simulink model "CG_5L_Inverter_simulinkblocks"  (R2024b)
settings: Solver=VariableStepAuto  StartTime=0.0  StopTime=0.6  RelTol=1e-3
libraries: spsIGBTDiodeLib x6, simulink x4, spsSeriesRLCBranchLib x4, spsDiodeLib x2, spsVoltageMeasurementLib x2, spsACVoltageSourceLib x1, spsDCVoltageSourceLib x1, spsCurrentMeasurementLib x1, spsRMSLib x1, sps_lib x1
settings Model: Creator=Kan  LastModifiedBy=DELL
settings SolverCC: AlgebraicLoopSolver=TrustRegion
settings DebuggingCC: ArithmeticOperatorsInVariantConditions=warning
settings SFSimCC: CustomCodeUndefinedFunction=UseInterfaceOnly
settings RTWCC: GPUComputeCapability=3.5

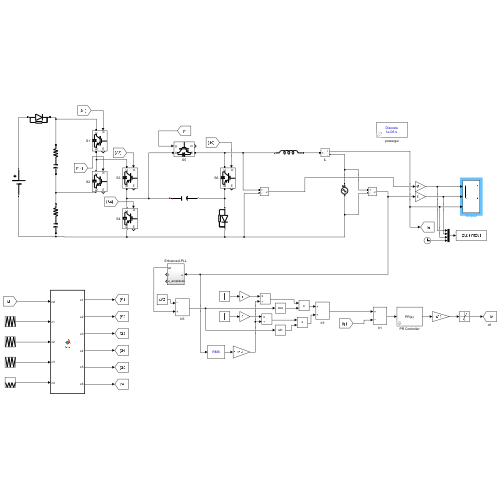
[thumbnail: Simulink's stored preview of the top-level diagram]
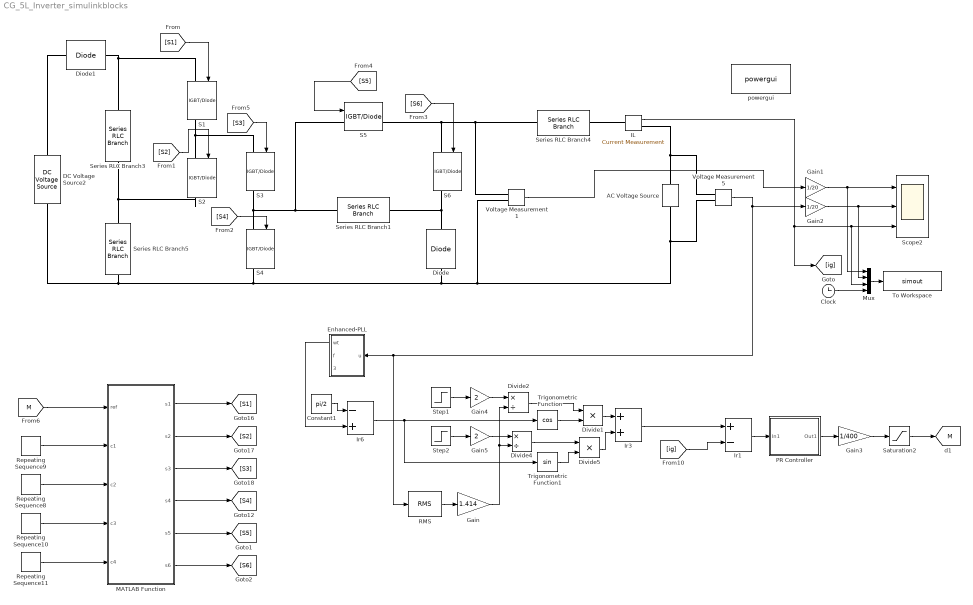
== system CG_5L_Inverter_simulinkblocks ==
  AC Voltage Source : spsACVoltageSourceLib/AC Voltage Source  Amplitude=325  Phase=0  Frequency=50  SampleTime=0  Measurements=None  BusType=swing  Pref=10e3  Qref=0  Qmin=-inf  Qmax=+inf
  Clock : Clock
  Constant1 : Constant  Value=pi/2
  DC Voltage Source2 : spsDCVoltageSourceLib/DC Voltage Source  Amplitude=400  Measurements=None
  Diode : spsDiodeLib/Diode  Ron=0.001  Lon=0  Vf=0.8  IC=0  UseSnubber=0  Rs=500000  Cs=250e-9  Measurements=off
  Diode1 : spsDiodeLib/Diode  Ron=0.001  Lon=0  Vf=0.8  IC=0  UseSnubber=0  Rs=500000  Cs=250e-9  Measurements=off
  Divide1 : Product  Inputs=**
  Divide2 : Product  Inputs=*/
  Divide4 : Product  Inputs=*/
  Divide5 : Product  Inputs=**
  Enhanced-PLL : Subsystem
  Gain : Gain  Gain=1.414
  Gain1 : Gain  Gain=1/20
  Gain2 : Gain  Gain=1/20
  Gain3 : Gain  Gain=1/400
  Gain4 : Gain  Gain=2
  Gain5 : Gain  Gain=2
  IL : spsCurrentMeasurementLib/Current Measurement  PhasorSimulation=off  OutputType=Complex  PSBequivalent=0
  Ir1 : Sum  Inputs=+-
  Ir3 : Sum
  Ir6 : Sum  Inputs=-+
  MATLAB Function : MATLAB Function  TreatAsAtomicUnit=on
  Mux : Mux
  PR Controller : Subsystem  mask(PR Controller){kp=5, kr=2000, f=50}
      mask prompts: kp "Proportional Gain (kp)"; kr "Resonant Gain (kr)"; f "Resonant Frequency (Hz)"
      mask help:
      | This block implements a Proportional Resonant Controller using transfer function kr*s / s^2+(2*pi*f)^2
      | It allows user to set the proportional gain (kp), resonant gain (kr) and resonant frequency in (Hz).
      |
      | Developed by Rodney Tan
      | Version 1.0 (Oct 2022)
      mask Display: disp('PR(s)');
  RMS : spsRMSLib/RMS  TrueRMS=on  Freq=50  RMSInit=120  Ts=0
  Repeating Sequence10 : simulink/Sources/Repeating Sequence  rep_seq_t=[0 1/20000 1/10000]  rep_seq_y=[0 -0.5 0]
  Repeating Sequence11 : simulink/Sources/Repeating Sequence  rep_seq_t=[0 1/20000 1/10000]  rep_seq_y=[-0.5 -1 -0.5]
  Repeating Sequence8 : simulink/Sources/Repeating Sequence  rep_seq_t=[0 1/20000 1/10000]  rep_seq_y=[0 0.5 0]
  Repeating Sequence9 : simulink/Sources/Repeating Sequence  rep_seq_t=[0 1/20000 1/10000]  rep_seq_y=[0.5 1 0.5]
  S{1..6} (6 alike) : spsIGBTDiodeLib/IGBT//Diode  Ron=1e-3  Rs=1e5  Cs=inf  Measurements=on
  Saturation2 : Saturate  UpperLimit=2  LowerLimit=-2  LinearizeAsGain=off
  Scope2 : Scope  NumInputPorts=3
  Series RLC Branch1 : spsSeriesRLCBranchLib/Series RLC Branch  LConnTagsString=__new0  RConnTagsString=__new0  BranchType=C  Resistance=1  Inductance=2e-3  SetiL0=off  InitialCurrent=0  Capacitance=4000e-6  Setx0=off  InitialVoltage=50  Measurements=None
  Series RLC Branch3 : spsSeriesRLCBranchLib/Series RLC Branch  LConnTagsString=__new0  RConnTagsString=__new0  BranchType=RC  Resistance=0.0002  Inductance=2e-3  SetiL0=off  InitialCurrent=0  Capacitance=2000e-6  Setx0=on  InitialVoltage=100  Measurements=None
  Series RLC Branch4 : spsSeriesRLCBranchLib/Series RLC Branch  LConnTagsString=__new0  RConnTagsString=__new0  BranchType=L  Resistance=0.0002  Inductance=6e-3  SetiL0=off  InitialCurrent=0  Capacitance=1e-6  Setx0=off  InitialVoltage=0  Measurements=None
  Series RLC Branch5 : spsSeriesRLCBranchLib/Series RLC Branch  LConnTagsString=__new0  RConnTagsString=__new0  BranchType=RC  Resistance=0.0002  Inductance=2e-3  SetiL0=off  InitialCurrent=0  Capacitance=2000e-6  Setx0=on  InitialVoltage=100  Measurements=None
  Step1 : Step  Time=0.3  Before=1000  After=0  SampleTime=0
  Step2 : Step  Time=0.3  After=1200  SampleTime=0
  To Workspace : ToWorkspace  VariableName=simout  SampleTime=-1
      settings: Save2DSignal=2-D array (concatenate along first dimension)
  Trigonometric Function : Trigonometry  Operator=cos
  Trigonometric Function1 : Trigonometry
  Voltage Measurement1 : spsVoltageMeasurementLib/Voltage Measurement  PhasorSimulation=off  OutputType=Complex  PSBequivalent=0
  Voltage Measurement5 : spsVoltageMeasurementLib/Voltage Measurement  PhasorSimulation=off  OutputType=Complex  PSBequivalent=0
  powergui : sps_lib/powergui  Priority=1  SimulationMode=Discrete  SampleTime=1e-6  frequency=60  Iterations=50  frequencyindice=0  Pbase=100e6  ErrMax=1e-4  UnitsV=kV  UnitsW=MW  buscounter=0  FunctionMessages=off  echomessages=off  EnableUseOfTLC=off  CurrentSourceSwitches=off  DisableSnubberDevices=off  DisableRonSwitches=off  DisableVfSwitches=off  DisplayEquations=off  AutomaticDiscreteSolvers=off  SolverType=Tustin/Backward Euler (TBE)  Interpol=off  ExternalGateDelay=off  methode=off  Ts=100  x0status=blocks  SPID=on  SwTol=0  HookPort=off  NonlinearTolerance=1e-4  nMaxIteration=100  ContinueOnMaxIteration=off  RestoreLinks=warning  ResistiveCurrentMeasurement=off  Frange=[0:2:500]  Ylog=off  Xlog=on  ShowGrid=off  save=off  variable=ZData  structure=0  ZoomFFT=off  StartTime=0.0  cycles=1  DisplayStyle=1  fundamental=60  FreqAxis=off  MaxFrequency=1000  frequencyindicesteady=1  RmsSteady=1  display=off
  tag scope: M=global
  wires:
  [S1] -> S1/1
  [S2] -> S2/1
  MATLAB Function/1(s1) -> [S1]
  MATLAB Function/4(s4) -> [S4]
  MATLAB Function/2(s2) -> [S2]
  [S3] -> S3/1
  [S4] -> S4/1
  [S5] -> S5/1
  [S6] -> S6/1
  MATLAB Function/5(s5) -> [S5]
  MATLAB Function/6(s6) -> [S6]
  Repeating Sequence11/1 -> MATLAB Function/5(c4)
  Repeating Sequence10/1 -> MATLAB Function/4(c3)
  Repeating Sequence8/1 -> MATLAB Function/3(c2)
  Repeating Sequence9/1 -> MATLAB Function/2(c1)
  Voltage Measurement1/1 -> Gain1/1
  Voltage Measurement5/1 -> RMS/1, Enhanced-PLL/1(u), Gain2/1
  Gain1/1 -> Mux/1, Scope2/1
  Gain2/1 -> Mux/2, Scope2/2
  Ir3/1 -> Ir1/1
  [ig] -> Ir1/2
  PR Controller/1(Out1) -> Gain3/1
  Saturation2/1 -> [M]
  Trigonometric Function1/1 -> Divide5/2
  Gain4/1 -> Divide2/1
  Divide5/1 -> Ir3/2
  Step2/1 -> Gain5/1
  Divide2/1 -> Divide1/1
  Constant1/1 -> Ir6/1
  Gain/1 -> Divide4/2, Divide2/2
  Gain5/1 -> Divide4/1
  Divide1/1 -> Ir3/1
  Step1/1 -> Gain4/1
  Trigonometric Function/1 -> Divide1/2
  RMS/1 -> Gain/1
  Ir6/1 -> Trigonometric Function1/1, Trigonometric Function/1
  Divide4/1 -> Divide5/1
  Enhanced-PLL/1(wt) -> Ir6/2
  Gain3/1 -> Saturation2/1
  Ir1/1 -> PR Controller/1(In1)
  IL/1 -> [ig], Mux/3, Scope2/3
  MATLAB Function/3(s3) -> [S3]
  [M] -> MATLAB Function/1(ref)
  Mux/1 -> To Workspace/1
  Clock/1 -> Mux/4
  connections:
  DC Voltage Source2/RConn1 -- Diode1/LConn1
  S5/RConn1 -- S6/LConn1 -- Series RLC Branch4/LConn1 -- Voltage Measurement1/LConn1
  S6/RConn1 -- Diode/LConn1 -- Series RLC Branch1/RConn1
  Voltage Measurement1/LConn2 -- DC Voltage Source2/LConn1 -- Series RLC Branch5/RConn1 -- S4/RConn1 -- Diode/RConn1 -- AC Voltage Source/LConn1 -- Voltage Measurement5/LConn2
  Series RLC Branch5/LConn1 -- S2/RConn1 -- Series RLC Branch3/RConn1
  S2/LConn1 -- S3/LConn1 -- S1/RConn1
  S4/LConn1 -- S5/LConn1 -- Series RLC Branch1/LConn1 -- S3/RConn1
  IL/LConn1 -- Series RLC Branch4/RConn1
  IL/RConn1 -- Voltage Measurement5/LConn1 -- AC Voltage Source/RConn1
  S1/LConn1 -- Diode1/RConn1 -- Series RLC Branch3/LConn1

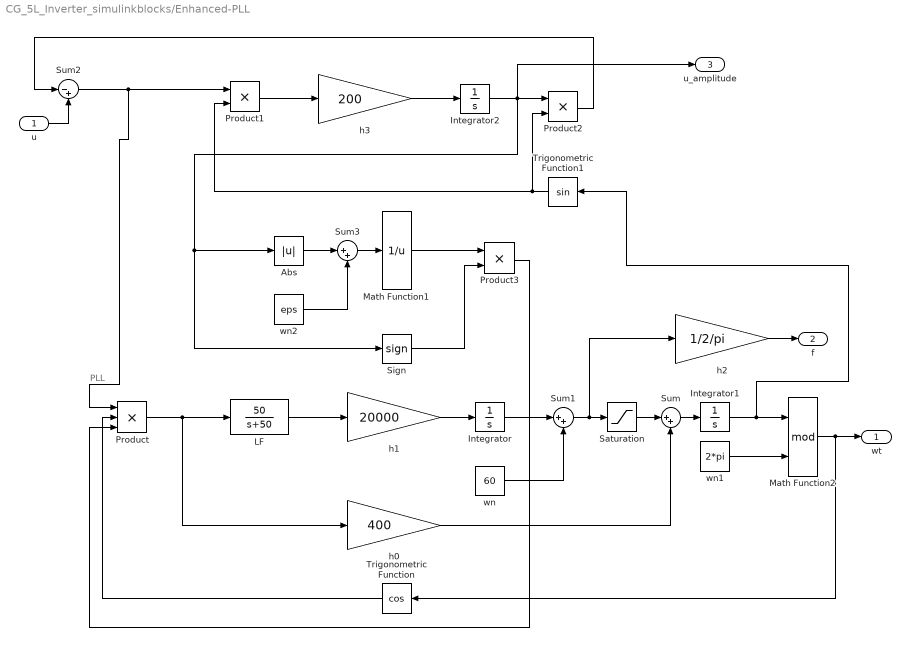
== system CG_5L_Inverter_simulinkblocks/Enhanced-PLL ==
  note: PLL
  u : Inport
  Abs : Abs  SaturateOnIntegerOverflow=off
  Integrator : Integrator
  Integrator1 : Integrator
  Integrator2 : Integrator
  LF : TransferFcn  Numerator=[50]  Denominator=[1 50]
  Math Function1 : Math  Operator=reciprocal  SignedPower=on
  Math Function2 : Math  Operator=mod  SignedPower=on
  Product : Product  Inputs=3
  Product1 : Product
  Product2 : Product
  Product3 : Product
  Saturation : Saturate  UpperLimit=2*pi*300  LowerLimit=2*pi*30
  Sign : Signum
  Sum : Sum  Inputs=|++
  Sum1 : Sum  Inputs=|++
  Sum2 : Sum  Inputs=|-+
  Sum3 : Sum  Inputs=|++
  Trigonometric Function : Trigonometry  Operator=cos
  Trigonometric Function1 : Trigonometry
  h0 : Gain  Gain=400
  h1 : Gain  Gain=20000
  h2 : Gain  Gain=1/2/pi
  h3 : Gain  Gain=200
  wn : Constant  Value=60
  wn1 : Constant  Value=2*pi
  wn2 : Constant  Value=eps
  wt : Outport
  f : Outport  Port=2
  u_amplitude : Outport  Port=3
  wires:
  h1/1 -> Integrator/1
  h0/1 -> Sum/2
  Product/1 -> h0/1, LF/1
  Sum/1 -> Integrator1/1
  Trigonometric Function/1 -> Product/2
  wn/1 -> Sum1/2
  Sum1/1 -> h2/1, Saturation/1
  Integrator/1 -> Sum1/1
  h2/1 -> f/1
  LF/1 -> h1/1
  Integrator1/1 -> Trigonometric Function1/1, Math Function2/1
  Math Function2/1 -> wt/1, Trigonometric Function/1
  wn1/1 -> Math Function2/2
  Trigonometric Function1/1 -> Product1/2, Product2/2
  Integrator2/1 -> u_amplitude/1, Sign/1, Abs/1, Product2/1
  h3/1 -> Integrator2/1
  Product1/1 -> h3/1
  Sum2/1 -> Product1/1, Product/1
  u/1 -> Sum2/2
  Product2/1 -> Sum2/1
  Abs/1 -> Sum3/1
  wn2/1 -> Sum3/2
  Sum3/1 -> Math Function1/1
  Math Function1/1 -> Product3/1
  Sign/1 -> Product3/2
  Product3/1 -> Product/3
  Saturation/1 -> Sum/1

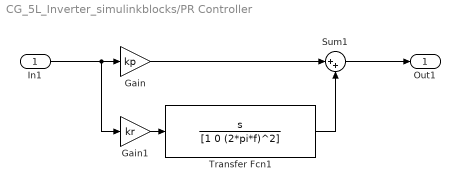
== system CG_5L_Inverter_simulinkblocks/PR Controller ==
  In1 : Inport
  Gain : Gain  Gain=kp
  Gain1 : Gain  Gain=kr
  Sum1 : Sum  Inputs=|++
  Transfer Fcn1 : TransferFcn  Numerator=[1 0]  Denominator=[1 0 (2*pi*f)^2]
  Out1 : Outport
  wires:
  Gain1/1 -> Transfer Fcn1/1
  Transfer Fcn1/1 -> Sum1/2
  In1/1 -> Gain1/1, Gain/1
  Sum1/1 -> Out1/1
  Gain/1 -> Sum1/1

== matlab function CG_5L_Inverter_simulinkblocks/MATLAB Function ==
  data: ref input; s1 output; c1 input; c2 input; c3 input; c4 input; s2 output; s3 output; s4 output; s5 output; s6 output
function [s1,s2,s3,s4,s5,s6] = fcn(ref,c1,c2,c3,c4)

if (ref>c1) % level 1
    s1=1;s2=0;s3=1;s4=0;s5=1;s6=0;
elseif (ref>c2 && ref <c1) % level 2
    s1=0;s2=1;s3=1;s4=0;s5=1;s6=0;
elseif (ref>c3 && ref <c2) % level 3
    s1=0;s2=0;s3=0;s4=1;s5=1;s6=0;
elseif (ref>c4 && ref <c3) % level 4
    s1=0;s2=1;s3=1;s4=0;s5=0;s6=1;
else % level 5
    s1=0;s2=0;s3=0;s4=1;s5=0;s6=1;

end
end
